simulink model "model"  (Simulink 7.7)
settings: Solver=ode3  StartTime=0.0  StopTime=3  FixedStep=0.05  RelTol=1e-3
undefined symbols (not defined in the file or in its folder): myspectre
settings Model: Creator=Eugeny  LastModifiedBy=ozisoft

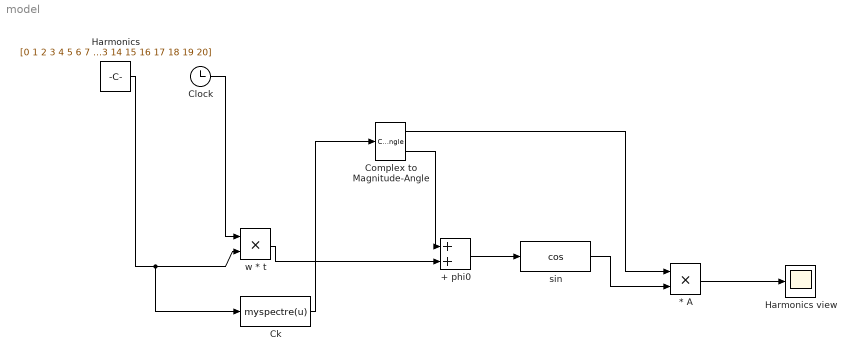
== system model ==
  * A : Product  RndMeth=Zero
  + phi0 : Sum
  Ck : MATLABFcn  MATLABFcn=myspectre(u)  OutputSignalType=complex
  Clock : Clock
      settings: Decimation=10
  Complex to Magnitude-Angle : ComplexToMagnitudeAngle
  Harmonics : Constant  Value=[0 1 2 3 4 5 6 7 8 9 10 11 12 13 14 15 16 17 18 19 20]
  Harmonics view : Scope
      settings: YMin=-0.5  YMax=0.5  SaveName=ScopeData2
  sin : MATLABFcn  MATLABFcn=cos
  w * t : Product  RndMeth=Zero
  wires:
  Ck/1 -> Complex to Magnitude-Angle/1
  Complex to Magnitude-Angle/1 -> * A/1
  Complex to Magnitude-Angle/2 -> + phi0/1
  Harmonics/1 -> w * t/2, Ck/1
  + phi0/1 -> sin/1
  w * t/1 -> + phi0/2
  sin/1 -> * A/2
  * A/1 -> Harmonics view/1
  Clock/1 -> w * t/1
